simulink model "state_estim_mdl"  (R2025b)
settings: Solver=VariableStepAuto  StartTime=0.0  StopTime=20  RelTol=1e-3
values from neighbouring files (symbols this model uses):
  ic = 0    [state_estim.m]
  L = acker(transpose(Ae), transpose(Ce),  -3 * [1 , 1, 1, 1, 1])    [state_estim.m]
  omega = 0.1 *2 * pi    (= 0.628318530718)    [state_estim.m]
  T = 1e-3    (= 0.001)    [state_estim.m]
undefined symbols (not defined in the file or in its folder): umax
libraries: simulink x2
settings Model: Creator=rapaja  LastModifiedBy=Predrag
settings SolverCC: AlgebraicLoopSolver=TrustRegion
settings DebuggingCC: UnconnectedInputMsg=warning  UnconnectedOutputMsg=warning  UnconnectedLineMsg=warning
settings ModelReferenceCC: EnableRefExpFcnMdlSchedulingChecks=on
settings RTWCC: GPUComputeCapability=3.5

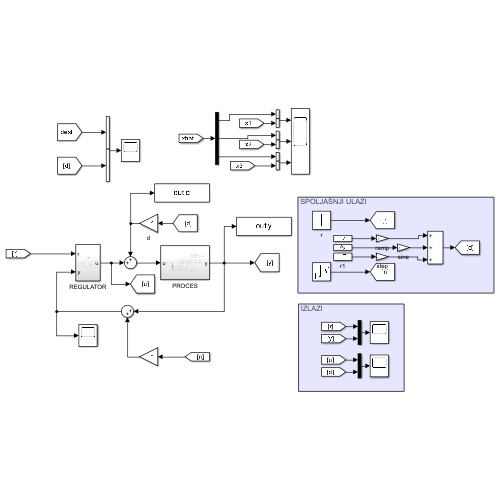
[thumbnail: Simulink's stored preview of the top-level diagram]
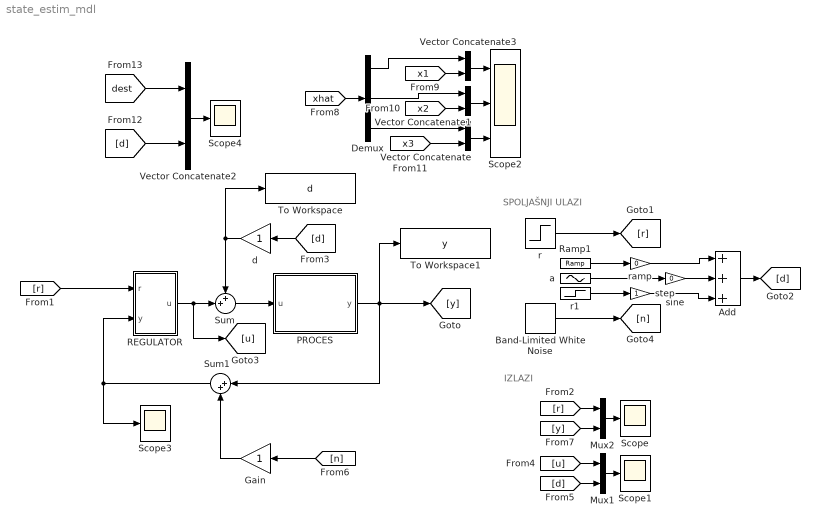
== system state_estim_mdl ==
  note: IZLAZI
  note: SPOLJAŠNJI ULAZI
  Add : Sum  Inputs=+++
  Band-Limited White Noise : simulink/Sources/Band-Limited White Noise  Cov=[0.00001]  Ts=T  seed=[23341]
  Demux : Demux  Outputs=3
  Gain : Gain
  Mux1 : Mux  Inputs=2
  Mux2 : Mux  Inputs=2
  PROCES : Subsystem
  REGULATOR : Subsystem
  Ramp1 : simulink/Sources/Ramp  slope=1  start=1  InitialOutput=0
  Scope{,1,3..4} (4 alike) : Scope
      Scope settings: ActiveDisplayYMinimum=-3.32902884493533  ActiveDisplayYMaximum=7.9291337351111064
      Scope1 settings: ActiveDisplayYMinimum=0.31655788074278879  ActiveDisplayYMaximum=1.0759380132508012
      Scope3 settings: ActiveDisplayYMinimum=-1.7038754366137421  ActiveDisplayYMaximum=1.8082472717172617  DataLoggingVariableName=ScopeData3
      Scope4 settings: ActiveDisplayYMinimum=-9.98491828429532  ActiveDisplayYMaximum=11.149469727890581  DataLoggingVariableName=ScopeData5
  Scope2 : Scope  NumInputPorts=3
      settings: ActiveDisplayYMinimum=-0.73428798733221023  ActiveDisplayYMaximum=6.73287010896767  DataLoggingVariableName=ScopeData2
  Sum : Sum  Inputs=++|
  Sum1 : Sum  Inputs=|++
  To Workspace : ToWorkspace  VariableName=d  SampleTime=-1
      settings: Save2DSignal=2-D array (concatenate along first dimension)
  To Workspace1 : ToWorkspace  VariableName=y  SampleTime=-1
      settings: Save2DSignal=2-D array (concatenate along first dimension)
  Vector Concatenate{,1..3} (4 alike) : Concatenate
  a : Sin  Frequency=omega  SampleTime=0
  d : Gain
  r : Step  SampleTime=0
  r1 : Step  Time=5  SampleTime=0
  ramp : Gain  Gain=0
  sine : Gain  Gain=0
  step : Gain
  wires:
  REGULATOR/1(u) -> Sum/2, [u]
  [d] -> d/1
  Band-Limited White Noise/1 -> [n]
  Gain/1 -> Sum1/2
  d/1 -> To Workspace/1, Sum/1
  [r] -> Mux2/1
  [y] -> Mux2/2
  Mux2/1 -> Scope/1
  Mux1/1 -> Scope1/1
  [u] -> Mux1/1
  [d] -> Mux1/2
  PROCES/1(y) -> To Workspace1/1, [y], Sum1/1
  Sum/1 -> PROCES/1(u)
  Sum1/1 -> Scope3/1, REGULATOR/2(y)
  r/1 -> [r]
  [n] -> Gain/1
  Vector Concatenate2/1 -> Scope4/1
  [d] -> Vector Concatenate2/2
  [dest] -> Vector Concatenate2/1
  [r] -> REGULATOR/1(r)
  [xhat] -> Demux/1
  Vector Concatenate/1 -> Scope2/3
  Demux/3 -> Vector Concatenate/1
  [x3] -> Vector Concatenate/2
  Vector Concatenate1/1 -> Scope2/2
  Demux/2 -> Vector Concatenate1/1
  [x2] -> Vector Concatenate1/2
  Vector Concatenate3/1 -> Scope2/1
  [x1] -> Vector Concatenate3/2
  Demux/1 -> Vector Concatenate3/1
  Ramp1/1 -> ramp/1
  a/1 -> sine/1
  r1/1 -> step/1
  sine/1 -> Add/2
  ramp/1 -> Add/1
  step/1 -> Add/3
  Add/1 -> [d]

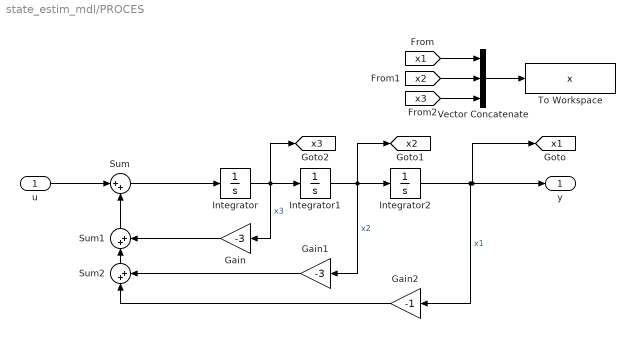
== system state_estim_mdl/PROCES ==
  u : Inport
  Gain : Gain  Gain=-3
  Gain1 : Gain  Gain=-3
  Gain2 : Gain  Gain=-1
  Integrator : Integrator  InitialCondition=ic
  Integrator1 : Integrator  InitialCondition=ic
  Integrator2 : Integrator  InitialCondition=ic
  Sum : Sum  Inputs=|++
  Sum1 : Sum  Inputs=|++
  Sum2 : Sum  Inputs=|++
  To Workspace : ToWorkspace  VariableName=x  SampleTime=-1
      settings: Save2DSignal=2-D array (concatenate along first dimension)
  Vector Concatenate : Concatenate  NumInputs=3
  y : Outport
  tag scope: x1=global, x2=global, x3=global
  wires:
  Integrator2/1 -> [x1], y/1, Gain2/1  "x1"
  Integrator1/1 -> [x2], Integrator2/1, Gain1/1  "x2"
  Integrator/1 -> [x3], Integrator1/1, Gain/1  "x3"
  u/1 -> Sum/1
  Sum/1 -> Integrator/1
  Gain/1 -> Sum1/2
  Sum1/1 -> Sum/2
  Sum2/1 -> Sum1/1
  Gain1/1 -> Sum2/2
  Gain2/1 -> Sum2/1
  [x1] -> Vector Concatenate/1
  [x2] -> Vector Concatenate/2
  [x3] -> Vector Concatenate/3
  Vector Concatenate/1 -> To Workspace/1

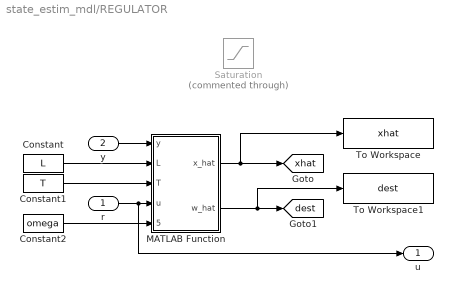
== system state_estim_mdl/REGULATOR ==
  r : Inport
  y : Inport  Port=2
  Constant : Constant  Value=L  VectorParams1D=off
  Constant1 : Constant  Value=T
  Constant2 : Constant  Value=omega
  MATLAB Function : MATLAB Function  TreatAsAtomicUnit=on
  Saturation : Saturate  Commented=through  UpperLimit=umax  LowerLimit=-umax
  To Workspace : ToWorkspace  VariableName=xhat  SampleTime=-1
      settings: Save2DSignal=2-D array (concatenate along first dimension)
  To Workspace1 : ToWorkspace  VariableName=dest  SampleTime=-1
      settings: Save2DSignal=2-D array (concatenate along first dimension)
  u : Outport
  tag scope: dest=global, xhat=global
  wires:
  y/1 -> MATLAB Function/1(y)
  Constant/1 -> MATLAB Function/2(L)
  Constant1/1 -> MATLAB Function/3(T)
  MATLAB Function/1(x_hat) -> To Workspace/1, [xhat]
  MATLAB Function/2(w_hat) -> To Workspace1/1, [dest]
  Constant2/1 -> MATLAB Function/5(omega)
  r/1 -> u/1, MATLAB Function/4(u)

== matlab function state_estim_mdl/REGULATOR/MATLAB Function ==
  settings: updateMethod=DISCRETE  sampleTime=T
  data: y input; x_hat output; L input; T input; u input; w_hat output; omega input
function [x_hat, w_hat] = fcn(y, L, T, u, omega)
persistent x1hat
persistent x2hat
persistent x3hat
persistent w1hat
persistent w2hat

if(isempty(x1hat))
    x1hat = 0;
end
if(isempty(x2hat))
    x2hat = 0;
end
if(isempty(x3hat))
    x3hat = 0;
end
if(isempty(w1hat))
    w1hat = 0;
end
if(isempty(w2hat))
    w2hat = 0;
end
e = y - x1hat;

x1hat_n = x1hat + T * (x2hat + L(1, 1) * e);
x2hat_n = x2hat + T * (x3hat + L(1, 2) * e);
x3hat_n = x3hat + T * (-3*x3hat - 3*x2hat -x1hat + u + w1hat + L(1, 3) * e);
w1hat_n = w1hat + T * ( w2hat + L(1, 4) * e);
w2hat_n = w2hat + T * (-omega^2 * w1hat +  L(1, 5) * e);

x1hat = x1hat_n;
x2hat = x2hat_n;
x3hat = x3hat_n;
w1hat = w1hat_n;
w2hat = w2hat_n;

x_hat = [x1hat, x2hat, x3hat];
w_hat = w1hat;
